simulink model "MKC_open_loop"  (R2025b)
settings: Solver=FixedStepAuto  StartTime=0.0  StopTime=time_sim  FixedStep=0.01  MaxStep=0.01  RelTol=1e-3
undefined symbols (not defined in the file): Amplitude, c, F_step, k, m, omega, v0, x0
settings Model: Creator=gianmarco  LastModifiedBy=gianmarco

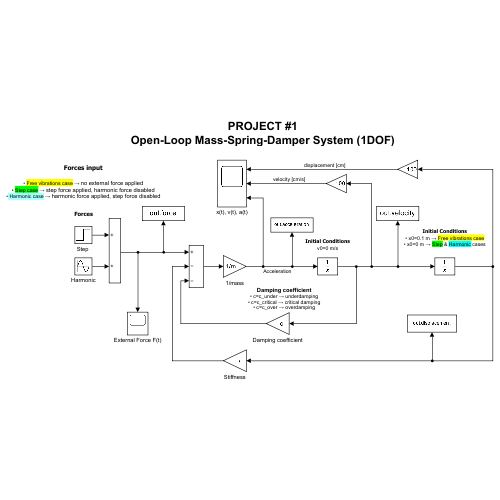
[thumbnail: Simulink's stored preview of the top-level diagram]
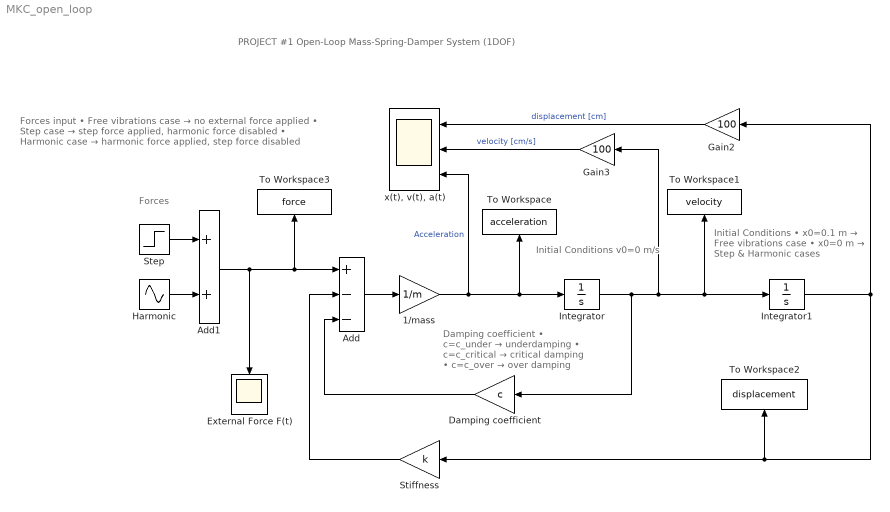
== system MKC_open_loop ==
  note: PROJECT #1
      | Open-Loop Mass-Spring-Damper System (1DOF)
  note: Forces
  note: Forces input
      |
      | • Free vibrations case → no external force applied
      | • Step case → step force applied, harmonic force disabled
      | • Harmonic case → harmonic force applied, step force disabled
  note: Damping coefficient
      | • c=c_under → underdamping
      | • c=c_critical → critical damping
      | • c=c_over → over damping
  note: Initial Conditions
      | v0=0 m/s
  note: Initial Conditions
      | • x0=0.1 m → Free vibrations case
      | • x0=0 m → Step & Harmonic cases
  1/mass : Gain  Gain=1/m
  Add : Sum  Inputs=+--
  Add1 : Sum
  Damping coefficient : Gain  Gain=c
  External Force F(t) : Scope
      settings: ActiveDisplayYMinimum=-1  ActiveDisplayYMaximum=1
  Gain2 : Gain  Gain=100
  Gain3 : Gain  Gain=100
  Harmonic : Sin  Amplitude=Amplitude  Frequency=omega  SampleTime=0
  Integrator : Integrator  InitialCondition=v0
  Integrator1 : Integrator  InitialCondition=x0
  "Step " : Step  Time=step  After=F_step  SampleTime=0
  Stiffness : Gain  Gain=k
  To Workspace : ToWorkspace  VariableName=acceleration  SampleTime=-1
  To Workspace1 : ToWorkspace  VariableName=velocity  SampleTime=-1
  To Workspace2 : ToWorkspace  VariableName=displacement  SampleTime=-1
  To Workspace3 : ToWorkspace  VariableName=force  SampleTime=-1
  "x(t), v(t), a(t)" : Scope  NumInputPorts=3
      settings: Title=Velocità  ActiveDisplayYMinimum=-50  ActiveDisplayYMaximum=40  YLabel=v(t) [cm/s]  DataLoggingVariableName=ScopeData4
  wires:
  1/mass/1 -> To Workspace/1, Integrator/1, "x(t), v(t), a(t)"/3  "Acceleration"
  Integrator/1 -> Damping coefficient/1, Gain3/1, Integrator1/1, To Workspace1/1
  Add/1 -> 1/mass/1
  Stiffness/1 -> Add/2
  Damping coefficient/1 -> Add/3
  Integrator1/1 -> Gain2/1, To Workspace2/1, Stiffness/1
  Add1/1 -> Add/1, To Workspace3/1, External Force F(t)/1
  "Step "/1 -> Add1/1
  Harmonic/1 -> Add1/2
  Gain2/1 -> "x(t), v(t), a(t)"/1  "displacement [cm]"
  Gain3/1 -> "x(t), v(t), a(t)"/2  "velocity [cm/s]"
